simulink model "Adaptive_BS"  (R2021b)
settings: Solver=FixedStepAuto  StartTime=0.0  StopTime=15.0  FixedStep=1e-3  RelTol=1e1
values from neighbouring files (symbols this model uses):
  Kd = diag([100 500 300 10 2 0.1])    [GuadagniControllore.m]
  lambda = diag([30 70 40 300 50 500])    [GuadagniControllore.m]
  m1 = L(1).m    [GuadagniControllore.m]
  m2 = L(2).m    [GuadagniControllore.m]
  m3 = L(3).m    [GuadagniControllore.m]
  m4 = L(4).m    [GuadagniControllore.m]
  m5 = L(5).m    [GuadagniControllore.m]
  m6 = L(6).m    [GuadagniControllore.m]
undefined symbols (not defined in the file or in its folder): B, l1, l2, l3, l4, l5, l6, q0, r, Spline
libraries: roblocks x3, robotcorelib x1, simulink x1
(part 5 of 5)

== matlab function Adaptive_BS/ABS control/parameters estimation ==
  data: Y input; dpi output; s input
function dpi = dyn_param(Y, s)
% Definisco una matrice definita positiva
R = diag([8.25 445 3960 8240 8390 44700]);
% Calcolo la dinamica di stima dei parametri
dpi = inv(R) * Y' * s;
